simulink model "DT_MotorCC_Multibody_w_vib_Vel_Control"  (R2023b)
settings: Solver=FixedStepAuto  StartTime=0.0  StopTime=10  FixedStep=0.0001  MaxStep=1e-3  RelTol=1e-3  AbsTol=1e-6
model workspace (MAT data in the model file):
  A = 5
  Frec = 1
  a = 1
values from neighbouring files (symbols this model uses):
  a_exp = 5.5449    [Parameters_MotorCC.m]
  a_pot = 70.434    [Parameters_MotorCC.m]
  b_exp = 0.0264    [Parameters_MotorCC.m]
  b_pot = 1.0329    [Parameters_MotorCC.m]
  J = (tau_m * K^2)/(Ra)    (= 0.000330907721143)    [Parameters_MotorCC.m]
  K_reductora = 1/30    (= 0.0333333333333)    [Parameters_MotorCC.m]
  K_taco = 8.07e-3    (= 0.00807)    [Parameters_MotorCC.m]
  PWM_sat = 8.78    [Parameters_MotorCC.m]
  sat_vib_max = 3.72    [Parameters_MotorCC.m]
  sat_vib_min = 0.4    [Parameters_MotorCC.m]
undefined symbols (not defined in the file or in its folder): smiData, X, Y, Z
libraries: fl_lib x40, nesl_utility x30, sm_lib x16, ee_lib x7, simulink x2, slpidlib x2, sdl_lib x1
(part 1 of 2)
settings Model: Creator=carlo  LastModifiedBy=carlo
settings SolverCC: EnableFixedStepZeroCrossing=on

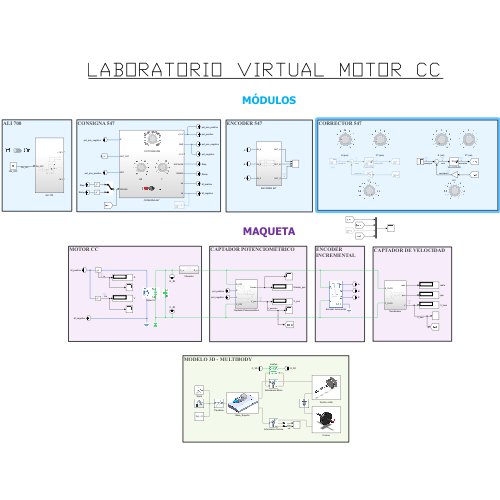
[thumbnail: Simulink's stored preview of the top-level diagram]
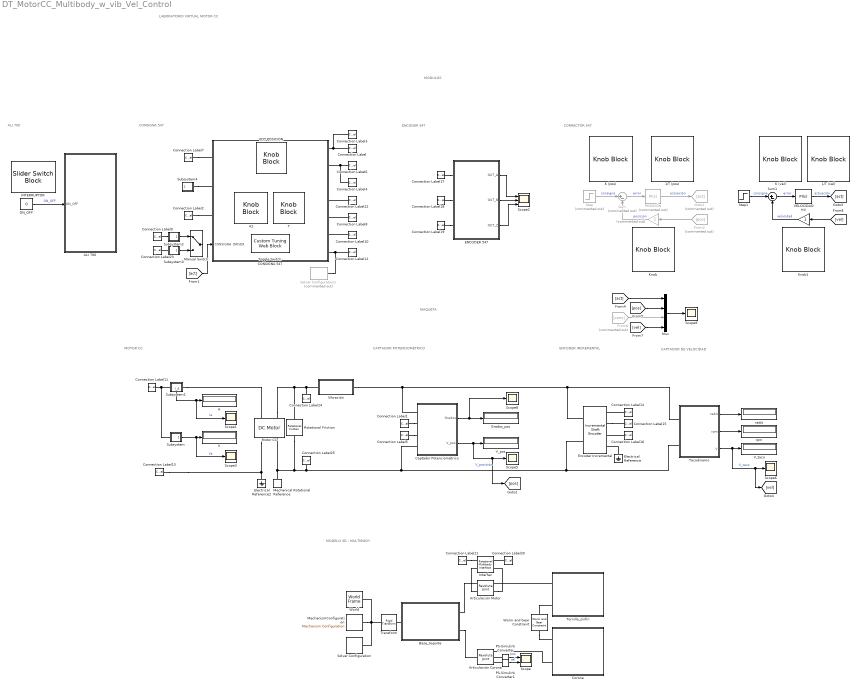
== system DT_MotorCC_Multibody_w_vib_Vel_Control ==
  note: MÓDULOS
  note: CORRECTOR 547
  note: CONSIGNA 547
  note: ENCODER 547
  note: ENCODER
      | INCREMENTAL
  note: CAPTADOR POTENCIOMÉTRICO
  note: MOTOR CC
  note: ALI 700
  note: MAQUETA
  note: LABORATORIO VIRTUAL MOTOR CC
  note: CAPTADOR DE VELOCIDAD
  note: MODELO 3D - MULTIBODY
  1/T (pos) : KnobBlock  LabelPosition=Hide  ScaleMax=10  TickInterval=1
  1/T (vel) : KnobBlock  LabelPosition=Hide  ScaleMax=10  TickInterval=1
  A : Display
  A2 : KnobBlock  LabelPosition=Hide  ScaleMax=10  TickInterval=1
  ALI 700 : Subsystem
  Articulación Corona : sm_lib/Joints/Revolute Joint  JointMode=Normal  SenseConstraintForce=off  SenseConstraintForceX=off  SenseConstraintForceY=off  SenseConstraintForceZ=off  SenseConstraintTorque=off  SenseConstraintTorqueX=off  SenseConstraintTorqueY=off  SenseConstraintTorqueZ=off  SenseTotalForce=off  SenseTotalForceX=off  SenseTotalForceY=off  SenseTotalForceZ=off  SenseTotalTorque=off  SenseTotalTorqueX=off  SenseTotalTorqueY=off  SenseTotalTorqueZ=off  CompositeWrenchDir=FollowerOnBase  CompositeWrenchFrame=BaseFrame  EquilibriumPosition=0  EquilibriumPositionUnits=deg  SpringStiffness=0  SpringStiffnessUnits=N*m/deg  DampingCoefficient=0  DampingCoefficientUnits=N*m/(deg/s)  TorqueActuationMode=NoTorque  MotionActuationMode=ComputedMotion  SensePosition=on  SenseVelocity=on  SenseAcceleration=off  SenseTorqueForce=off  SenseLowerLimitTorqueForce=off  SenseUpperLimitTorqueForce=off  LowerLimitSpecify=off  LowerLimitBound=-90  LowerLimitBoundUnits=deg  LowerLimitStiffness=1e4  LowerLimitStiffnessUnits=N*m/deg  LowerLimitDamping=10  LowerLimitDampingUnits=N*m/(deg/s)  LowerLimitTransitionRegionWidth=0.1  LowerLimitTransitionRegionWidthUnits=deg  UpperLimitSpecify=off  UpperLimitBound=90  UpperLimitBoundUnits=deg  UpperLimitStiffness=1e4  UpperLimitStiffnessUnits=N*m/deg  UpperLimitDamping=10  UpperLimitDampingUnits=N*m/(deg/s)  UpperLimitTransitionRegionWidth=0.1  UpperLimitTransitionRegionWidthUnits=deg  PositionTargetSpecify=on  PositionTargetPriority=Low  PositionTargetValue=smiData.RevoluteJoint(2).Rz.Pos  PositionTargetValueUnits=deg  VelocityTargetSpecify=off  VelocityTargetPriority=High  VelocityTargetValue=0  VelocityTargetValueUnits=deg/s
  Articulación Motor : sm_lib/Joints/Revolute Joint  JointMode=Normal  SenseConstraintForce=off  SenseConstraintForceX=off  SenseConstraintForceY=off  SenseConstraintForceZ=off  SenseConstraintTorque=off  SenseConstraintTorqueX=off  SenseConstraintTorqueY=off  SenseConstraintTorqueZ=off  SenseTotalForce=off  SenseTotalForceX=off  SenseTotalForceY=off  SenseTotalForceZ=off  SenseTotalTorque=off  SenseTotalTorqueX=off  SenseTotalTorqueY=off  SenseTotalTorqueZ=off  CompositeWrenchDir=FollowerOnBase  CompositeWrenchFrame=BaseFrame  EquilibriumPosition=0  EquilibriumPositionUnits=deg  SpringStiffness=0  SpringStiffnessUnits=N*m/deg  DampingCoefficient=0  DampingCoefficientUnits=N*m/(deg/s)  TorqueActuationMode=InputTorque  MotionActuationMode=ComputedMotion  SensePosition=off  SenseVelocity=on  SenseAcceleration=off  SenseTorqueForce=off  SenseLowerLimitTorqueForce=off  SenseUpperLimitTorqueForce=off  LowerLimitSpecify=off  LowerLimitBound=-90  LowerLimitBoundUnits=deg  LowerLimitStiffness=1e4  LowerLimitStiffnessUnits=N*m/deg  LowerLimitDamping=10  LowerLimitDampingUnits=N*m/(deg/s)  LowerLimitTransitionRegionWidth=0.1  LowerLimitTransitionRegionWidthUnits=deg  UpperLimitSpecify=off  UpperLimitBound=90  UpperLimitBoundUnits=deg  UpperLimitStiffness=1e4  UpperLimitStiffnessUnits=N*m/deg  UpperLimitDamping=10  UpperLimitDampingUnits=N*m/(deg/s)  UpperLimitTransitionRegionWidth=0.1  UpperLimitTransitionRegionWidthUnits=deg  PositionTargetSpecify=on  PositionTargetPriority=Low  PositionTargetValue=smiData.RevoluteJoint(1).Rz.Pos  PositionTargetValueUnits=deg  VelocityTargetSpecify=off  VelocityTargetPriority=High  VelocityTargetValue=0  VelocityTargetValueUnits=deg/s
  Base_Soporte : Subsystem
      mask Display: image('Base.png');
  CONSIGNA 547 : Subsystem
      settings: PortSchema="{\"entries\":[{\"content\":{\"sides\":[{\"content\":{\"connectorIds\":[\"LConn1\",\"LConn2\",\"LConn3\",\"In1\"]},\"type\":\"ConnectorPlacement.EquallySpacedRectSide\",\"uuid\":\"4a8cfb57-dab5-486b-a591-dc2fea0d0b24\"},{\"content\":{\"connectorIds\":[\"RConn1\",\"RConn2\",\"RConn3\",\"RConn4\",\"RConn5\",\"RConn6\",\"RConn7\"],\"side\":\"RIGHT\"},\"type\":\"ConnectorPlacement.EquallySpacedRectSide\",\"uuid\":\"c23f5fb5-28b8-45c6-932c-b7e70ba2c44b\"},{\"content\":{\"side\":\"TOP\"},\"type\":\"ConnectorPlacement.EquallySpacedRectSide\",\"uuid\":\"d5136a80-57f8-4106-bad8-2d611f5e0ad7\"}]},\"type\":\"ConnectorPlacement.EquallySpacedConnector\",\"uuid\":\"b8a23e2e-242e-4702-9d69-57328d2e8c40\"}],\"packageUris\":[\"http://schema.mathworks.com/mf0/Connector/R2020b\"],\"version\":\"1.0\"}"
  Captador Potenciométrico : Subsystem
  Connection Label : ConnectionLabel  Label=pot_positivo
  Connection Label1 : ConnectionLabel  Label=pot_positivo
  Connection Label10 : ConnectionLabel  Label=M_positivo
  Connection Label11 : ConnectionLabel  Label=M_positivo
  Connection Label12 : ConnectionLabel  Label=M_negativo
  Connection Label13 : ConnectionLabel  Label=M_negativo
  Connection Label14 : ConnectionLabel  Label=A
  Connection Label15 : ConnectionLabel  Label=B
  Connection Label16 : ConnectionLabel  Label=Z
  Connection Label17 : ConnectionLabel  Label=A
  Connection Label18 : ConnectionLabel  Label=B
  Connection Label19 : ConnectionLabel  Label=Z
  Connection Label2 : ConnectionLabel  Label=pot_pos_positivo
  Connection Label20 : ConnectionLabel  Label=R_3D
  Connection Label21 : ConnectionLabel  Label=C_3D
  Connection Label22 : ConnectionLabel  Label=Step
  Connection Label23 : ConnectionLabel  Label=Ramp
  Connection Label24 : ConnectionLabel  Label=R_3D
  Connection Label25 : ConnectionLabel  Label=C_3D
  Connection Label3 : ConnectionLabel  Label=pot_pos_positivo
  Connection Label4 : ConnectionLabel  Label=pot_negativo
  Connection Label5 : ConnectionLabel  Label=pot_negativo
  Connection Label6 : ConnectionLabel  Label=pot_pos_negativo
  Connection Label7 : ConnectionLabel  Label=pot_pos_negativo
  Connection Label8 : ConnectionLabel  Label=Ramp
  Connection Label9 : ConnectionLabel  Label=Step
  Corona : Subsystem
      mask Display: image('Corona.png');
  ENCODER 547 : Subsystem
  Electrical Reference : fl_lib/Electrical/Electrical Elements/Electrical Reference
  Electrical Reference2 : fl_lib/Electrical/Electrical Elements/Electrical Reference
  Encoder Incremental : ee_lib/Sensors & Transducers/Incremental Shaft Encoder  NPulse=50  Vm=5 V  angle0=0 deg
      settings: InternalSimscapePortConfiguration="{\"Bottom\":[],\"Left\":[{\"id\":\"R\",\"label\":\"R\",\"type\":\"foundation.mechanical.rotational.rotational\"},{\"id\":\"C\",\"label\":\"C\",\"type\":\"foundation.mechanical.rotational.rotational\"}],\"Right\":[{\"id\":\"A\",\"label\":\"A\",\"type\":\"foundation.electrical.electrical\"},{\"id\":\"B\",\"label\":\"B\",\"type\":\"foundation.electrical.electrical\"},{\"id\":\"Z\",\"label\":\"Z\",\"type\":\"foundation.electrical.electrical\"},{\"id\":\"GND\",\"label\":\"REF\",\"type\":\"foundation.electrical.electrical\"}],\"Top\":[]}"
  From2 : From  Commented=on  GotoTag=pos
  From6 : From  Commented=on  GotoTag=cons
  Goto1 : Goto  Commented=on  GotoTag=act
  Grados_pos : Display
  HP : Gain  Commented=on
  HV : Gain
  INTERRUPTOR : SliderSwitchBlock  LabelPosition=Hide
      settings: Values={{'Off', 'On'}, [0 1]}
  Interfaz : fl_lib/Mechanical/Multibody Interfaces/Rotational Multibody Interface
  K (pos) : KnobBlock  LabelPosition=Hide  ScaleMax=10  TickInterval=1
  K (vel) : KnobBlock  LabelPosition=Hide  ScaleMax=10  TickInterval=1
  Knob : KnobBlock  LabelPosition=Hide  ScaleMax=1  TickInterval=0.1
  Knob1 : KnobBlock  LabelPosition=Hide  ScaleMax=2  TickInterval=0.2
  Manual Switch : ManualSwitch
  Mechanical Rotational Reference : fl_lib/Mechanical/Rotational Elements/Mechanical Rotational Reference
  MechanismConfiguration : sm_lib/Utilities/Mechanism Configuration  UniformGravity=None  GravityVector=[0 -9.80665 0]  GravityVectorUnits=m/s^2  LinearizationDelta=0.001  JointModeTransitionNonlinearIterations=2
  Motor CC : ee_lib/Electromechanical/Brushed Motors/DC Motor  field_option=ee.enum.field_option.pm  Rf=100 Ohm  Lf=1 H  Laf=0.15 H  If0=0 A  parameterization=ee.enum.dcparam_option.circuit_param  Ra=Ra Ohm  La=La mH  emf_or_torque=ee.enum.emf_or_torque.kv  Kv=K V*s/rad  Ki=6.876e-4 N*m/A  T_stall=0.24e-3 N*m  w_max=19100 rpm  w_rated=15000 rpm  P_rated=0.08 W  V_rated=1.5 V  lam_param=ee.enum.lam_param.damping  i_noload=0.069 A  V_i_noload=6.96 V  J=J kg*m^2  lam=0 N*m*s/rad  speed0=0 rpm  enable_fault_armature=simscape.enum.onoff.off  rev_faulted=1 / 3  G_faulted_armature=1e-5 S  fault_trigger_armature=ee.enum.faults.faultTrigger.temporal  t_fault_armature=1 s  max_permissible_current_armature=inf A  t_fail_on_current_armature=1 s  enable_fault_field=simscape.enum.onoff.off  G_faulted_field=1e-5 S  fault_trigger_field=ee.enum.faults.faultTrigger.temporal  t_fault_field=1 s  max_permissible_current_field=inf A  t_fail_on_current_field=1 s  fault_action=simscape.enum.assert.action.none  alpha=3.93e-3 1/K  Tmeas=25 degC  thermal_mass=100 J/K  initial_temperature=25 degC
  Mux : Mux
  ON_OFF : Constant  Value=0
  POSICIÓN : slpidlib/PID Controller  Commented=on  Controller=PI  Form=Ideal  TimeDomain=Continuous-time  UseExternalTs=off  SampleTime=-1  IntegratorMethod=Forward Euler  FilterMethod=Forward Euler  ControllerParametersSource=internal  P=2  I=1  UseKiTs=off  D=0  N=100  UseFilter=on  TunerSelectOption=Transfer Function Based (PID Tuner App)  InitialConditionSource=internal  InitialConditionForIntegrator=0  InitialConditionForFilter=0  DifferentiatorICPrevScaledInput=0  ExternalReset=none  TrackingMode=off  Kt=1  LimitOutput=on  SatLimitsSource=internal  UpperSaturationLimit=10  LowerSaturationLimit=-10  LinearizeAsGain=on  AntiWindupMode=back-calculation  Kb=1  LimitIntegrator=off  UpperIntegratorSaturationLimit=inf  LowerIntegratorSaturationLimit=-inf  POutMin=[]  POutMax=[]  IOutMin=[]  IOutMax=[]  DOutMin=[]  DOutMax=[]  NOutMin=[]  NOutMax=[]  SumOutMin=[]  SumOutMax=[]  SaturationOutMin=[]  SaturationOutMax=[]  PParamMin=[]  PParamMax=[]  IParamMin=[]  IParamMax=[]  DParamMin=[]  DParamMax=[]  NParamMin=[]  NParamMax=[]  KbParamMin=[]  KbParamMax=[]  KtParamMin=[]  KtParamMax=[]  KbOutMin=[]  KbOutMax=[]  KtOutMin=[]  KtOutMax=[]  IntegratorOutMin=[]  IntegratorOutMax=[]  FilterOutMin=[]  FilterOutMax=[]  SumI1OutMin=[]  SumI1OutMax=[]  SumI2OutMin=[]  SumI2OutMax=[]  SumI3OutMin=[]  SumI3OutMax=[]  SumI4OutMin=[]  SumI4OutMax=[]  SumDOutMin=[]  SumDOutMax=[]  DifferentiatorOutMin=[]  DifferentiatorOutMax=[]  FilterDiffOutCoefMin=[]  FilterDiffOutCoefMax=[]  ReciprocalOutMin=[]  ReciprocalOutMax=[]  SumDenOutMin=[]  SumDenOutMax=[]  SumNumOutMin=[]  SumNumOutMax=[]  DivideOutMin=[]  DivideOutMax=[]  UdiffTsProdOutMin=[]  UdiffTsProdOutMax=[]  NTsProdOutMin=[]  NTsProdOutMax=[]  UintegralTsProdOutMin=[]  UintegralTsProdOutMax=[]  UngainTsProdOutMin=[]  UngainTsProdOutMax=[]  ClampingZeroOutDataTypeStr=Inherit: Inherit via back propagation  ClampingZeroOutMin=[]  ClampingZeroOutMax=[]  FilterDenConstantOutDataTypeStr=Inherit: Inherit via back propagation  FilterDenConstantOutMin=[]  FilterDenConstantOutMax=[]  PCopyOutDataTypeStr=Inherit: Inherit via back propagation  PCopyOutMin=[]  PCopyOutMax=[]  NCopyOutDataTypeStr=Inherit: Inherit via back propagation  NCopyOutMin=[]  NCopyOutMax=[]  IntegratorContinuousStateAttributes=''  IntegratorStateMustResolveToSignalObject=off  IntegratorRTWStateStorageClass=Auto  FilterContinuousStateAttributes=''  FilterStateMustResolveToSignalObject=off  FilterRTWStateStorageClass=Auto  ParallelPVariant=Passthrough  IdealPVariant=InternalParameters  IVariant=InternalParameters  DVariant=Disabled  IntegratorVariant=Continuous  SatVariant=Enabled  AWVariant=BackCalculation  PCopyVariant=Disabled  TRVariant=Disabled  FdbkBlocksVariant=Forward  IdealPFdbkVariant=Disabled  SatFdbkVariant=Disabled  DerivativeFilterVariant=Disabled  NVariant=Disabled  NCopyVariant=Disabled_SignalSpec  FilterICVariant=Disabled  IntegratorICVariant=InternalICs  ExternalResetVariant=Disabled  TRSumVariant=Passthrough  SumFdbkVariant=Disabled  SumVariant=Sum_PI  TsampFilterVariant=InternalTs  TsampNgainVariant=Passthrough  TsampIntegralVariant=Disabled_SignalSpec  ExternalSaturationOutDataTypeStr=Inherit: Same as second input
  POT POSICIÓN : KnobBlock  LabelPosition=Hide  ScaleMax=360  TickInterval=20
  PS-Simulink Converter : nesl_utility/PS-Simulink Converter  PhysicalDomain=network_engine_domain  SubClassName=ps_output  LeftPortType=input  RightPortType=output  PseudoPeriodic=off  Frequencies=[]  VectorFormat=inherit  Unit=inherit  AffineConversion=off
  PS-Simulink Converter1 : nesl_utility/PS-Simulink Converter  PhysicalDomain=network_engine_domain  SubClassName=ps_output  LeftPortType=input  RightPortType=output  PseudoPeriodic=off  Frequencies=[]  VectorFormat=inherit  Unit=inherit  AffineConversion=off
  Rotational Friction : fl_lib/Mechanical/Rotational Elements/Rotational Friction  brkwy_trq=Tf N*m  brkwy_vel=0.1 rad/s  Col_trq=Tf N*m  visc_coef=B N*m*s/rad  w_specify=off  w_priority=None  w=0 rad/s  w_nominal_specify=off  w_nominal_unit=rad/s  w_nominal_value=1  t_specify=off  t_priority=None  t=0 N*m  t_nominal_specify=off  t_nominal_unit=N*m  t_nominal_value=1
  Scope : Scope  NumInputPorts=2
  Scope{1,3,5..6,8..9} (6 alike) : Scope
  Scope2 : Scope  NumInputPorts=3
  Solver Configuration : nesl_utility/Solver Configuration  PhysicalDomain=network_engine_domain  SubClassName=solver  LeftPortType=input  RightPortType=generic  Tones=[]  Harmonics=[]  SimulateNoise=off  Profile=off  UseLocalSampling=off  EnableSwitchedLinearOptims=on  FrequencyDomain=off  UseCCode=off  RelTol=0.001  AbsTol=0.001  MinStep=1e-09  ToWorkspace=off  RevertToSquareIcSolve=off  NumHomotopyIterations=100  PhasorMode=off  PhasorModeNumHarmonics=1  ConsistencySolver=NEWTON_XTOL_AFTER_FTOL  IndexReductionMethod=DerivativeReplacement  DoDC=off  ResidualTolerance=1e-09  ConsistencyTolSource=GLOBAL  ConsistencyAbsTol=0.001  ConsistencyRelTol=0.001  ConsistencyTolFactor=0.001  UseLocalSolver=off  LocalSolverChoice=NE_BACKWARD_EULER_ADVANCER  ResolveIndetEquations=on  FunctionEvalNumThread=1  LocalSolverSampleTime=0.001  DoFixedCost=off  MaxNonlinIter=3  MaxModeIter=2  ComputeImpulses=off  ImpulseIterations=2  LinearAlgebra=auto  LinearAlgebraNumThread=0  EquationFormulation=NE_TIME_EF  DelaysMemoryBudget=1024  AutomaticFiltering=on  FilteringTimeConstant=0.001  PartitionStorageMethod=AS_NEEDED  PartitionMemoryBudget=1024  PartitionMethod=ROBUST  MultibodyUseLocalSolver=off  MultibodyLocalSolverChoice=ODE3  MultibodyLocalSolverSampleTime=0.001
  Solver Configuration1 : nesl_utility/Solver Configuration  Commented=on  PhysicalDomain=network_engine_domain  SubClassName=solver  LeftPortType=input  RightPortType=generic  Tones=[]  Harmonics=[]  SimulateNoise=off  Profile=off  UseLocalSampling=off  EnableSwitchedLinearOptims=on  FrequencyDomain=off  UseCCode=off  RelTol=0.001  AbsTol=0.001  MinStep=1e-09  ToWorkspace=off  RevertToSquareIcSolve=off  NumHomotopyIterations=100  PhasorMode=off  PhasorModeNumHarmonics=1  ConsistencySolver=NEWTON_XTOL_AFTER_FTOL  IndexReductionMethod=DerivativeReplacement  DoDC=off  ResidualTolerance=1e-09  ConsistencyTolSource=GLOBAL  ConsistencyAbsTol=0.001  ConsistencyRelTol=0.001  ConsistencyTolFactor=0.001  UseLocalSolver=off  LocalSolverChoice=NE_BACKWARD_EULER_ADVANCER  ResolveIndetEquations=on  FunctionEvalNumThread=1  LocalSolverSampleTime=0.001  DoFixedCost=off  MaxNonlinIter=3  MaxModeIter=2  ComputeImpulses=off  ImpulseIterations=2  LinearAlgebra=auto  LinearAlgebraNumThread=0  EquationFormulation=NE_TIME_EF  DelaysMemoryBudget=1024  AutomaticFiltering=on  FilteringTimeConstant=0.001  PartitionStorageMethod=AS_NEEDED  PartitionMemoryBudget=1024  PartitionMethod=ROBUST  MultibodyUseLocalSolver=off  MultibodyLocalSolverChoice=ODE1  MultibodyLocalSolverSampleTime=0.001
  Step : Step  Commented=on  Time=5  Before=2  After=5  SampleTime=0
  Step1 : Step  Time=0  After=4  SampleTime=0
  Subsystem : Subsystem
      mask Display: disp('V');
  Subsystem1 : Subsystem
      settings: PortSchema="{\"entries\":[{\"content\":{\"sides\":[{\"content\":{\"connectorIds\":[\"LConn1\"]},\"type\":\"ConnectorPlacement.EquallySpacedRectSide\",\"uuid\":\"5f01206e-22b9-410b-acd2-df307548d4ec\"},{\"content\":{\"connectorIds\":[\"RConn1\"],\"side\":\"RIGHT\"},\"type\":\"ConnectorPlacement.EquallySpacedRectSide\",\"uuid\":\"8e9acb11-d78e-4e8a-8f36-3c08acadde04\"},{\"content\":{\"side\":\"TOP\"},\"type\":\"ConnectorPlacement.EquallySpacedRectSide\",\"uuid\":\"00b5443d-0936-4894-9d98-e1c6e581c2ec\"},{\"content\":{\"connectorIds\":[\"Out1\"],\"side\":\"BOTTOM\"},\"type\":\"ConnectorPlacement.EquallySpacedRectSide\",\"uuid\":\"fd0e1e3c-499b-4234-81ad-1a1f6c7863b2\"}]},\"type\":\"ConnectorPlacement.EquallySpacedConnector\",\"uuid\":\"3f6111df-7811-4c91-97b5-222f2bb21be8\"}],\"packageUris\":[\"http://schema.mathworks.com/mf0/Connector/R2020b\"],\"version\":\"1.0\"}"
      mask Display: disp('A');
  Subsystem2 : Subsystem
      mask Display: disp('V');
  Subsystem3 : Subsystem
      mask Display: disp('V');
  Subsystem4 : Subsystem
      mask Display: disp('V');
  Sum : Sum  Commented=on  Inputs=|+-
  Sum1 : Sum  Inputs=|+-
  T : KnobBlock  LabelPosition=Hide  ScaleMax=10  TickInterval=1
  Tacodinamo : Subsystem
  Toggle Switch : CustomTuningWebBlock  LabelPosition=Hide  ShowInitialText=on  Configuration="{\"components\":[{\"name\":\"CustomSwitchStateComponent\",\"settings\":{\"position\":[0,0,1,1],\"showAllLabels\":1,\"states\":[{\"HitRegion\":{\"position\":[0.03,0,0.518,1]},\"Image\":{\"position\":[0.24928571428571428,0,1,0.5014285714285714],\"size\":[1,0.5014285714285714],\"src\":\"data:image\\/svg+xml;base64,PHN2ZyB4bWxucz0iaHR0cDovL3d3dy53My5vcmcvMjAwMC9zdmciIHhtbG5zOnhsaW5rPSJodHRwOi8vd3d3LnczLm9yZy8xOTk5L3hsaW5rIiB2aWV3Qm94PSIwIDAgMzguMDQgMTUwIj48ZGVmcz48c3R5bGU+LmNscy0xe2ZpbGw6dXJsKCNyYWRpYWwtZ3JhZGllbnQpO30uY2xzLTJ7ZmlsbDp1cmwoI3JhZGlhbC1ncmFkaWVudC0yKTt9LmNscy0ze2ZpbGw6dXJsKCNXaGl0ZV9CbGFjayk7fS5jbHMtNHtmaWxsOnVybCgjcmFkaWFsLWdyYWRpZW50LTMpO30uY2xzLTV7ZmlsbDojNWI1YjViO30uY2xzLTZ7ZmlsbDp1cmwoI3Jh ...(+3556 chars)\",\"srcOrientation\":\"Right\"},\"Label\":{\"color\":[0.5019607843137255,0.5019607843137255,0.5019607843137255],\"icon\":{\"size\":[0,0],\"src\":[],\"srcOrientation\":\"Right\"},\"iconPlacement\":\"left\",\"opacity\":1,\"position\":[0.5,0.07999999999999996],\"show\":true,\"text\":{\"content\":\"+\",\"font\":\"Helvetica\",\"fontSize\":26}},\"Value\":1},{\"HitRegion\":{\"position\":[0,0.5,0.5,1]},\"Image\":{\"position\":[0.24928571428571428,0,1,0.5014285714285714],\"size\":[1,0.5014285714285714],\"src\":\"data:image\\/svg+xml;base64,PHN2ZyB4bWxucz0iaHR0cDovL3d3dy53My5vcmcvMjAwMC9zdmciIHhtbG5zOnhsaW5rPSJodHRwOi8vd3d3LnczLm9yZy8xOTk5L3hsaW5rIiB2aWV3Qm94PSIwIDAgMzguMDQgMTUwIj48ZGVmcz48c3R5bGU+LmNscy0xe2ZpbGw6dXJsKCNyYWRpYWwtZ3JhZGllbnQpO30uY2xzLTJ7ZmlsbDp1cmwoI3JhZGlhbC1ncmFkaWVudC0yKTt9LmNscy0ze2ZpbGw6dXJsKCNXaGl0ZV9CbGFjayk7fS5jbHMtNHtmaWxsOnVybCgjcmFkaWFsLWdyYWRpZW50LTMpO30uY2xzLTV7ZmlsbDojNWI1YjViO30uY2xzLTZ7ZmlsbDp1cmwoI3Jh ...(+3628 chars)\",\"srcOrientation\":\"Right\"},\"Label\":{\"color\":[0,0,0],\"icon\":{\"size\":[0,0],\"src\":[],\"srcOrientation\":\"Right\"},\"iconPlacement\":\"left\",\"opacity\":1,\"position\":[0.5,0.9],\"show\":true,\"text\":{\"content\":\"-\",\"font\":\"Helvetica\",\"fontSize\":26}},\"Value\":-1}]}},{\"name\":\"BackgroundImageComponent\",\"settings\":{\"image\":{\"size\":[70,135],\"src\":\"default\",\"srcOrientation\":\"Right\"},\"position\":[0,0,1,1],\"scaleMode\":\"0\"}},{\"name\":\"ForegroundImageComponent\",\"settings\":{\"image\":{\"size\":[0,0],\"src\":\"default\",\"srcOrientation\":[]},\"isForeground\":1,\"position\":[0,0,1,1],\"scaleMode\":\"0\"}}],\"settings\":{\"BindingType\":\"param\",\"backgroundColor\":[0,0,0],\"backgroundOffset\":0.14,\"fixedAspectRatio\":\"on\",\"foregroundColor\":[0,0,0],\"showBackgroundColor\":false,\"variant\":\"toggle\",\"version\":\"R2023a\"},\"type\":\"Switch\"}"
  Tornillo_sinfín : Subsystem
      mask Display: image('Tornillo_sinfin.png');
  Transform : sm_lib/Frames and Transforms/Rigid Transform  TranslationMethod=Cartesian  TranslationStandardOffset=0  TranslationStandardOffsetUnits=m  TranslationStandardAxis=+Z  TranslationCartesianOffset=smiData.RigidTransform(5).translation  TranslationCartesianOffsetUnits=mm  TranslationROffset=0  TranslationROffsetUnits=m  TranslationZOffset=0  TranslationZOffsetUnits=m  TranslationThetaOffset=0  TranslationThetaOffsetUnits=deg  RotationMethod=ArbitraryAxis  RotationAngleUnits=rad  RotationStandardAxis=+Z  RotationAngle=smiData.RigidTransform(5).angle  RotationArbitraryAxis=smiData.RigidTransform(5).axis  FollAlignAxisA=+X  BaseAlignAxisA=+Y  FollAlignAxisB=+Y  BaseAlignAxisB=+Z  RotationSequenceAxes=FollowerAxes  RotationSequence=XYX  RotationSequenceAngles=[0 0 0]  RotationSequenceAnglesUnits=deg  RotationMatrix=[1 0 0; 0 1 0; 0 0 1]  Quaternion=[1 0 0 0]
  V : Display
  VELOCIDAD : slpidlib/PID Controller  Controller=PI  Form=Ideal  TimeDomain=Continuous-time  UseExternalTs=off  SampleTime=-1  IntegratorMethod=Forward Euler  FilterMethod=Forward Euler  ControllerParametersSource=internal  P=2  I=1  UseKiTs=off  D=0  N=100  UseFilter=on  TunerSelectOption=Transfer Function Based (PID Tuner App)  InitialConditionSource=internal  InitialConditionForIntegrator=0  InitialConditionForFilter=0  DifferentiatorICPrevScaledInput=0  ExternalReset=none  TrackingMode=off  Kt=1  LimitOutput=on  SatLimitsSource=internal  UpperSaturationLimit=10  LowerSaturationLimit=-10  LinearizeAsGain=on  AntiWindupMode=back-calculation  Kb=1  LimitIntegrator=off  UpperIntegratorSaturationLimit=inf  LowerIntegratorSaturationLimit=-inf  POutMin=[]  POutMax=[]  IOutMin=[]  IOutMax=[]  DOutMin=[]  DOutMax=[]  NOutMin=[]  NOutMax=[]  SumOutMin=[]  SumOutMax=[]  SaturationOutMin=[]  SaturationOutMax=[]  PParamMin=[]  PParamMax=[]  IParamMin=[]  IParamMax=[]  DParamMin=[]  DParamMax=[]  NParamMin=[]  NParamMax=[]  KbParamMin=[]  KbParamMax=[]  KtParamMin=[]  KtParamMax=[]  KbOutMin=[]  KbOutMax=[]  KtOutMin=[]  KtOutMax=[]  IntegratorOutMin=[]  IntegratorOutMax=[]  FilterOutMin=[]  FilterOutMax=[]  SumI1OutMin=[]  SumI1OutMax=[]  SumI2OutMin=[]  SumI2OutMax=[]  SumI3OutMin=[]  SumI3OutMax=[]  SumI4OutMin=[]  SumI4OutMax=[]  SumDOutMin=[]  SumDOutMax=[]  DifferentiatorOutMin=[]  DifferentiatorOutMax=[]  FilterDiffOutCoefMin=[]  FilterDiffOutCoefMax=[]  ReciprocalOutMin=[]  ReciprocalOutMax=[]  SumDenOutMin=[]  SumDenOutMax=[]  SumNumOutMin=[]  SumNumOutMax=[]  DivideOutMin=[]  DivideOutMax=[]  UdiffTsProdOutMin=[]  UdiffTsProdOutMax=[]  NTsProdOutMin=[]  NTsProdOutMax=[]  UintegralTsProdOutMin=[]  UintegralTsProdOutMax=[]  UngainTsProdOutMin=[]  UngainTsProdOutMax=[]  ClampingZeroOutDataTypeStr=Inherit: Inherit via back propagation  ClampingZeroOutMin=[]  ClampingZeroOutMax=[]  FilterDenConstantOutDataTypeStr=Inherit: Inherit via back propagation  FilterDenConstantOutMin=[]  FilterDenConstantOutMax=[]  PCopyOutDataTypeStr=Inherit: Inherit via back propagation  PCopyOutMin=[]  PCopyOutMax=[]  NCopyOutDataTypeStr=Inherit: Inherit via back propagation  NCopyOutMin=[]  NCopyOutMax=[]  IntegratorContinuousStateAttributes=''  IntegratorStateMustResolveToSignalObject=off  IntegratorRTWStateStorageClass=Auto  FilterContinuousStateAttributes=''  FilterStateMustResolveToSignalObject=off  FilterRTWStateStorageClass=Auto  ParallelPVariant=Passthrough  IdealPVariant=InternalParameters  IVariant=InternalParameters  DVariant=Disabled  IntegratorVariant=Continuous  SatVariant=Enabled  AWVariant=BackCalculation  PCopyVariant=Disabled  TRVariant=Disabled  FdbkBlocksVariant=Forward  IdealPFdbkVariant=Disabled  SatFdbkVariant=Disabled  DerivativeFilterVariant=Disabled  NVariant=Disabled  NCopyVariant=Disabled_SignalSpec  FilterICVariant=Disabled  IntegratorICVariant=InternalICs  ExternalResetVariant=Disabled  TRSumVariant=Passthrough  SumFdbkVariant=Disabled  SumVariant=Sum_PI  TsampFilterVariant=InternalTs  TsampNgainVariant=Passthrough  TsampIntegralVariant=Disabled_SignalSpec  ExternalSaturationOutDataTypeStr=Inherit: Same as second input
  V_pos : Display
  V_taco : Display
  Vibración : Subsystem
  World : sm_lib/Frames and Transforms/World Frame
  Worm and Gear Constraint : sm_lib/Gears and Couplings/Gears/Worm and Gear Constraint  WormDirection=RightHand  WormLeadAngle=10  WormLeadAngleUnits=deg  SpecificationMethod=CenterDistanceRatio  CenterDistance=3.35  CenterDistanceUnits=cm  Ratio=30  WormRadius=10  WormRadiusUnits=cm  GearRadius=10  GearRadiusUnits=cm
  rad/s : Display
  rpm : Display
  wires:
  Subsystem/1(output) -> Scope3/1, V/1  "Va"
  Captador Potenciométrico/2(V_pos) -> [pos], Scope5/1, V_pos/1  "V_posición"
  ON_OFF/1 -> ALI 700/1(ON_OFF)  "ON_OFF"
  ENCODER 547/3(OUT_Z) -> Scope2/3
  ENCODER 547/2(OUT_B) -> Scope2/2
  Sum/1 -> POSICIÓN/1  "error"
  POSICIÓN/1 -> Goto1/1  "actuación"
  Sum1/1 -> VELOCIDAD/1  "error"
  VELOCIDAD/1 -> [act]  "actuación"
  HV/1 -> Sum1/2  "velocidad"
  HP/1 -> Sum/2  "posicion"
  Step1/1 -> Sum1/1  "consigna"
  [vel] -> HV/1
  ENCODER 547/1(OUT_A) -> Scope2/1
  Subsystem1/1(I_A) -> Scope1/1, A/1  "Ia"
  Subsystem2/1(output) -> Manual Switch/1
  Subsystem3/1(output) -> Manual Switch/2
  Tacodinamo/3(V) -> [vel], Scope6/1, V_taco/1  "V_taco"
  Tacodinamo/1(rad/s) -> rad/s/1
  Tacodinamo/2(rpm) -> rpm/1
  Captador Potenciométrico/1(Grados) -> Scope8/1, Grados_pos/1
  PS-Simulink Converter1/1 -> Scope/2  "vel"
  PS-Simulink Converter/1 -> Scope/1  "pos"
  [act] -> CONSIGNA 547/1(CONSIGNA  DRIVER)
  Step/1 -> Sum/1  "consigna"
  Mux/1 -> Scope9/1
  [act] -> Mux/1
  [pos] -> Mux/2
  From6/1 -> Mux/3
  [vel] -> Mux/4
  From2/1 -> HP/1
  connections:
  Tacodinamo/LConn2 -- Encoder Incremental/LConn2 -- Captador Potenciométrico/LConn4 -- Connection Label25/LConn1 -- Rotational Friction/RConn1 -- Mechanical Rotational Reference/LConn1 -- Motor CC/RConn2
  Subsystem1/LConn1 -- Connection Label11/LConn1 -- Subsystem/LConn1
  Connection Label14/LConn1 -- Encoder Incremental/RConn1
  Encoder Incremental/RConn2 -- Connection Label15/LConn1
  Connection Label/LConn1 -- Connection Label3/LConn1 -- CONSIGNA 547/RConn1
  Motor CC/RConn1 -- Connection Label13/LConn1 -- Electrical Reference2/LConn1
  Connection Label17/LConn1 -- ENCODER 547/LConn1
  Connection Label18/LConn1 -- ENCODER 547/LConn2
  Connection Label19/LConn1 -- ENCODER 547/LConn3
  Electrical Reference/LConn1 -- Encoder Incremental/RConn4
  Connection Label16/LConn1 -- Encoder Incremental/RConn3
  Connection Label22/LConn1 -- CONSIGNA 547/RConn4
  Connection Label8/LConn1 -- CONSIGNA 547/RConn5
  Subsystem1/RConn1 -- Motor CC/LConn1
  Connection Label9/LConn1 -- Subsystem2/LConn1
  Subsystem3/LConn1 -- Connection Label23/LConn1
  Motor CC/LConn2 -- Vibración/LConn1 -- Connection Label24/LConn1 -- Rotational Friction/LConn1
  World/RConn1 -- MechanismConfiguration/RConn1 -- Transform/LConn1 -- Solver Configuration/RConn1
  PS-Simulink Converter/LConn1 -- Articulación Corona/RConn2
  PS-Simulink Converter1/LConn1 -- Articulación Corona/RConn3
  Worm and Gear Constraint/LConn1 -- Tornillo_sinfín/LConn2
  Base_Soporte/LConn1 -- Transform/RConn1
  Base_Soporte/RConn1 -- Articulación Motor/LConn1
  Base_Soporte/RConn2 -- Articulación Corona/LConn1
  Tornillo_sinfín/LConn1 -- Articulación Motor/RConn1
  Worm and Gear Constraint/RConn1 -- Corona/LConn1
  Corona/LConn2 -- Articulación Corona/RConn1
  Connection Label20/LConn1 -- Interfaz/RConn2
  Connection Label21/LConn1 -- Interfaz/LConn2
  Subsystem4/LConn1 -- CONSIGNA 547/LConn2
  Connection Label7/LConn1 -- CONSIGNA 547/LConn1
  Connection Label2/LConn1 -- CONSIGNA 547/LConn3
  Articulación Motor/RConn2 -- Interfaz/RConn1
  Interfaz/LConn1 -- Articulación Motor/LConn2
  Connection Label4/LConn1 -- Connection Label6/LConn1 -- CONSIGNA 547/RConn2
  Connection Label5/LConn1 -- Captador Potenciométrico/LConn3
  Connection Label1/LConn1 -- Captador Potenciométrico/LConn2
  Connection Label10/LConn1 -- CONSIGNA 547/RConn6
  CONSIGNA 547/RConn7 -- Solver Configuration1/RConn1 -- Connection Label12/LConn1
  Vibración/RConn1 -- Captador Potenciométrico/LConn1 -- Encoder Incremental/LConn1 -- Tacodinamo/LConn1

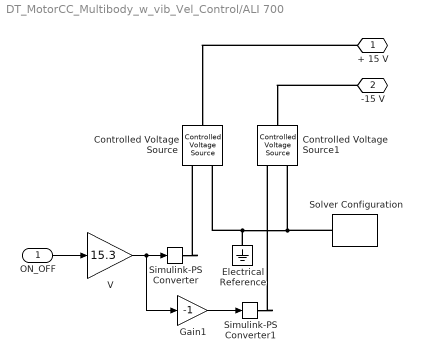
== system DT_MotorCC_Multibody_w_vib_Vel_Control/ALI 700 ==
  ON_OFF : Inport
  Controlled Voltage Source : fl_lib/Electrical/Electrical Sources/Controlled Voltage Source
  Controlled Voltage Source1 : fl_lib/Electrical/Electrical Sources/Controlled Voltage Source
  Electrical Reference : fl_lib/Electrical/Electrical Elements/Electrical Reference
  Gain1 : Gain  Gain=-1
  Simulink-PS Converter : nesl_utility/Simulink-PS Converter  PhysicalDomain=network_engine_domain  SubClassName=ps_input  LeftPortType=input  RightPortType=output  PseudoPeriodic=off  Frequencies=[]  NoiseDistribution=none  NoiseParameters=[]  Unit=V  AffineConversion=off  FilteringAndDerivatives=provide  SimscapeFilterOrder=1  InputFilterTimeConstant=0.001  UdotUserProvided=0
  Simulink-PS Converter1 : nesl_utility/Simulink-PS Converter  PhysicalDomain=network_engine_domain  SubClassName=ps_input  LeftPortType=input  RightPortType=output  PseudoPeriodic=off  Frequencies=[]  NoiseDistribution=none  NoiseParameters=[]  Unit=1  AffineConversion=off  FilteringAndDerivatives=provide  SimscapeFilterOrder=1  InputFilterTimeConstant=0.001  UdotUserProvided=0
  Solver Configuration : nesl_utility/Solver Configuration  PhysicalDomain=network_engine_domain  SubClassName=solver  LeftPortType=input  RightPortType=generic  Tones=[]  Harmonics=[]  SimulateNoise=off  Profile=off  UseLocalSampling=off  EnableSwitchedLinearOptims=on  FrequencyDomain=off  UseCCode=off  RelTol=0.001  AbsTol=0.001  MinStep=1e-09  ToWorkspace=off  RevertToSquareIcSolve=off  NumHomotopyIterations=100  PhasorMode=off  PhasorModeNumHarmonics=1  ConsistencySolver=NEWTON_XTOL_AFTER_FTOL  IndexReductionMethod=DerivativeReplacement  DoDC=off  ResidualTolerance=1e-09  ConsistencyTolSource=GLOBAL  ConsistencyAbsTol=0.001  ConsistencyRelTol=0.001  ConsistencyTolFactor=0.001  UseLocalSolver=off  LocalSolverChoice=NE_BACKWARD_EULER_ADVANCER  ResolveIndetEquations=on  FunctionEvalNumThread=1  LocalSolverSampleTime=0.001  DoFixedCost=off  MaxNonlinIter=3  MaxModeIter=2  ComputeImpulses=off  ImpulseIterations=2  LinearAlgebra=auto  LinearAlgebraNumThread=0  EquationFormulation=NE_TIME_EF  DelaysMemoryBudget=1024  AutomaticFiltering=on  FilteringTimeConstant=0.001  PartitionStorageMethod=AS_NEEDED  PartitionMemoryBudget=1024  PartitionMethod=ROBUST  MultibodyUseLocalSolver=off  MultibodyLocalSolverChoice=ODE1  MultibodyLocalSolverSampleTime=0.001
  V : Gain  Gain=15.3
  + 15 V : PMIOPort  Side=Right
  -15 V : PMIOPort  Port=2  Side=Right
  wires:
  ON_OFF/1 -> V/1
  Gain1/1 -> Simulink-PS Converter1/1
  V/1 -> Gain1/1, Simulink-PS Converter/1
  connections:
  Electrical Reference/LConn1 -- Solver Configuration/RConn1 -- Controlled Voltage Source1/RConn2 -- Controlled Voltage Source/RConn2
  + 15 V/RConn1 -- Controlled Voltage Source/LConn1
  -15 V/RConn1 -- Controlled Voltage Source1/LConn1
  Simulink-PS Converter/RConn1 -- Controlled Voltage Source/RConn1
  Simulink-PS Converter1/RConn1 -- Controlled Voltage Source1/RConn1

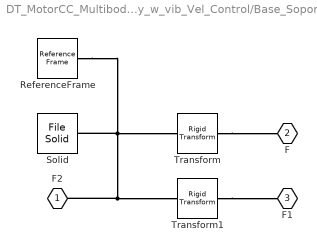
== system DT_MotorCC_Multibody_w_vib_Vel_Control/Base_Soporte ==
  ReferenceFrame : sm_lib/Frames and Transforms/Reference Frame
  Solid : sm_lib/Body Elements/File Solid  ExtGeomFileName=Base.STEP  UnitType=FromFile  ExtGeomFileUnits=m  StepReaderType=HEX  ExportConvexHullGeometry=off  InertiaType=Custom  Mass=smiData.Solid(2).mass  MassUnits=kg  CenterOfMass=smiData.Solid(2).CoM  CenterOfMassUnits=mm  MomentsOfInertia=smiData.Solid(2).MoI  MomentsOfInertiaUnits=kg*mm^2  ProductsOfInertia=smiData.Solid(2).PoI  ProductsOfInertiaUnits=kg*mm^2  BasedOnType=DensityFromFile  Density=1000  DensityUnits=kg/m^3  DoExposeReferenceFrame=on  SerializedFrames=<Frames/>  GraphicType=FromGeometry  MarkerShape=Sphere  MarkerSize=10  GraphicVisPropType=SimpleVisualProperties  GraphicDiffuseColor=smiData.Solid(2).color  GraphicSpecularColor=[0.5 0.5 0.5 1.0]  GraphicAmbientColor=[0.15 0.15 0.15 1.0]  GraphicEmissiveColor=[0.0 0.0 0.0 1.0]  GraphicShininess=75  GraphicOpacity=smiData.Solid(2).opacity
  Transform : sm_lib/Frames and Transforms/Rigid Transform  TranslationMethod=Cartesian  TranslationStandardOffset=0  TranslationStandardOffsetUnits=m  TranslationStandardAxis=+Z  TranslationCartesianOffset=smiData.RigidTransform(1).translation  TranslationCartesianOffsetUnits=mm  TranslationROffset=0  TranslationROffsetUnits=m  TranslationZOffset=0  TranslationZOffsetUnits=m  TranslationThetaOffset=0  TranslationThetaOffsetUnits=deg  RotationMethod=ArbitraryAxis  RotationAngleUnits=rad  RotationStandardAxis=+Z  RotationAngle=smiData.RigidTransform(1).angle  RotationArbitraryAxis=smiData.RigidTransform(1).axis  FollAlignAxisA=+X  BaseAlignAxisA=+Y  FollAlignAxisB=+Y  BaseAlignAxisB=+Z  RotationSequenceAxes=FollowerAxes  RotationSequence=XYX  RotationSequenceAngles=[0 0 0]  RotationSequenceAnglesUnits=deg  RotationMatrix=[1 0 0; 0 1 0; 0 0 1]  Quaternion=[1 0 0 0]
  Transform1 : sm_lib/Frames and Transforms/Rigid Transform  TranslationMethod=Cartesian  TranslationStandardOffset=0  TranslationStandardOffsetUnits=m  TranslationStandardAxis=+Z  TranslationCartesianOffset=smiData.RigidTransform(3).translation  TranslationCartesianOffsetUnits=mm  TranslationROffset=0  TranslationROffsetUnits=m  TranslationZOffset=0  TranslationZOffsetUnits=m  TranslationThetaOffset=0  TranslationThetaOffsetUnits=deg  RotationMethod=ArbitraryAxis  RotationAngleUnits=rad  RotationStandardAxis=+Z  RotationAngle=smiData.RigidTransform(3).angle  RotationArbitraryAxis=smiData.RigidTransform(3).axis  FollAlignAxisA=+X  BaseAlignAxisA=+Y  FollAlignAxisB=+Y  BaseAlignAxisB=+Z  RotationSequenceAxes=FollowerAxes  RotationSequence=XYX  RotationSequenceAngles=[0 0 0]  RotationSequenceAnglesUnits=deg  RotationMatrix=[1 0 0; 0 1 0; 0 0 1]  Quaternion=[1 0 0 0]
  F2 : PMIOPort  Side=Left
  F : PMIOPort  Port=2  Side=Right
  F1 : PMIOPort  Port=3  Side=Right
  connections:
  ReferenceFrame/RConn1 -- Solid/RConn1 -- Transform1/LConn1 -- F2/RConn1 -- Transform/LConn1
  Transform/RConn1 -- F/RConn1
  Transform1/RConn1 -- F1/RConn1
